simulink model "zustandsRegler"  (R2019b)
settings: Solver=FixedStepAuto  StartTime=0.0  StopTime=7  FixedStep=0.001  MaxStep=1e-3  RelTol=1e-3
values from neighbouring files (symbols this model uses):
  ausgangsVektor_cT = [0,1]    [initm.m]
  eingangsVektor_b = [0;2.63]    [initm.m]
  K = lqr(system_s, [1,0;0,1], 1)    [initm.m]
  systemMatrix_A = [0,2.63;0,0]    [initm.m]

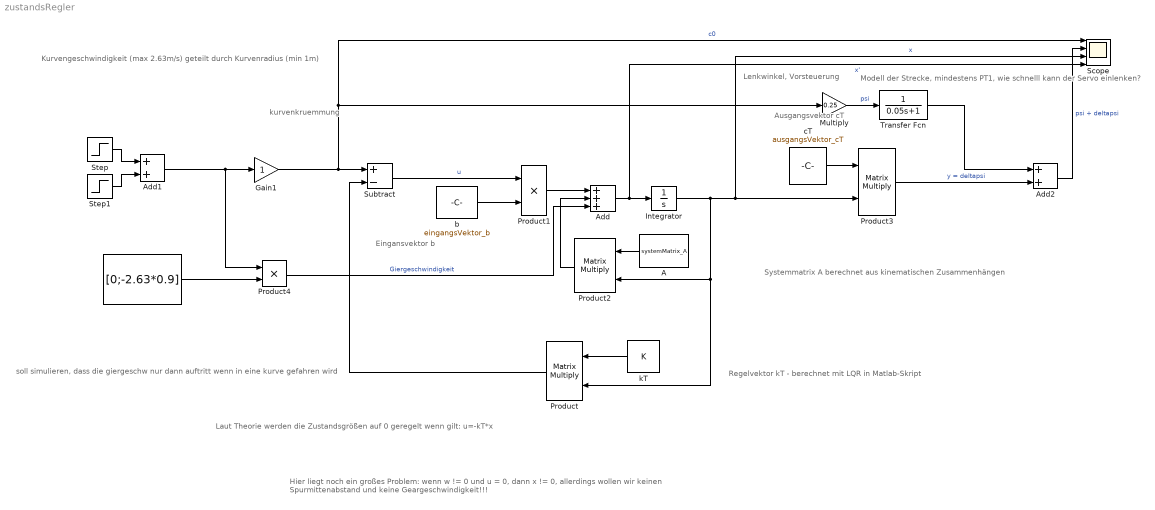
== system zustandsRegler ==
  note: Modell der Strecke, mindestens PT1, wie schnelll kann der Servo einlenken?
  note: Lenkwinkel, Vorsteuerung
  note: kurvenkruemmung
  note: soll simulieren, dass die giergeschw nur dann auftritt wenn in eine kurve gefahren wird
  note: Laut Theorie werden die Zustandsgrößen auf 0 geregelt wenn gilt: u=-kT*x
  note: Hier liegt noch ein großes Problem: wenn w != 0 und u = 0, dann x != 0, allerdings wollen wir keinen Spurmittenabstand und keine Geargeschwindigkeit!!!
  note: Ausgangsvektor cT
  note: Eingansvektor b
  note: Systemmatrix A berechnet aus kinematischen Zusammenhängen
  note: Regelvektor kT - berechnet mit LQR in Matlab-Skript
  note: Kurvengeschwindigkeit (max 2.63m/s) geteilt durch Kurvenradius (min 1m)
  " " : Constant  Value=[0;-2.63*0.9]
  A : Constant  Value=systemMatrix_A  VectorParams1D=off
  Add : Sum  Inputs=+++
  Add1 : Sum
  Add2 : Sum
  Gain1 : Gain
  Integrator : Integrator
  Multiply : Gain  Gain=0.25
  Product : Product  Multiplication=Matrix(*)
  Product1 : Product
  Product2 : Product  Multiplication=Matrix(*)
  Product3 : Product  Multiplication=Matrix(*)
  Product4 : Product
  Scope : Scope  NumInputPorts=4
  Step : Step  SampleTime=0
  Step1 : Step  Time=5  After=-1  SampleTime=0
  Subtract : Sum  Inputs=+-
  Transfer Fcn : TransferFcn  Denominator=[0.05 1]
  b : Constant  Value=eingangsVektor_b  VectorParams1D=off
  cT : Constant  Value=ausgangsVektor_cT  VectorParams1D=off
  kT : Constant  Value=K  VectorParams1D=off
  wires:
  Add/1 -> Scope/4, Integrator/1  "x'"
  Product1/1 -> Add/1
  Product2/1 -> Add/2
  b/1 -> Product1/2
  A/1 -> Product2/1
  kT/1 -> Product/1
  Integrator/1 -> Scope/3, Product3/2, Product/2, Product2/2  "x"
  cT/1 -> Product3/1
  Subtract/1 -> Product1/1  "u"
  Product/1 -> Subtract/2
  Add1/1 -> Product4/1, Gain1/1
  " "/1 -> Product4/2
  Gain1/1 -> Scope/1, Multiply/1, Subtract/1  "c0"
  Product4/1 -> Add/3  "Giergeschwindigkeit"
  Product3/1 -> Add2/2  "y = deltapsi"
  Multiply/1 -> Transfer Fcn/1  "psi"
  Add2/1 -> Scope/2  "psi + deltapsi"
  Step/1 -> Add1/1
  Step1/1 -> Add1/2
  Transfer Fcn/1 -> Add2/1
